simulink model "TemperatureConverter"  (R2024a)
settings: Solver=VariableStepAuto  StartTime=0.0  StopTime=10.0  RelTol=1e-3
values from neighbouring files (symbols this model uses):
  C = input(prompt)    [TemperatureConverter_TrialRun.m]
settings Model: Creator=ammaa  LastModifiedBy=ammaa

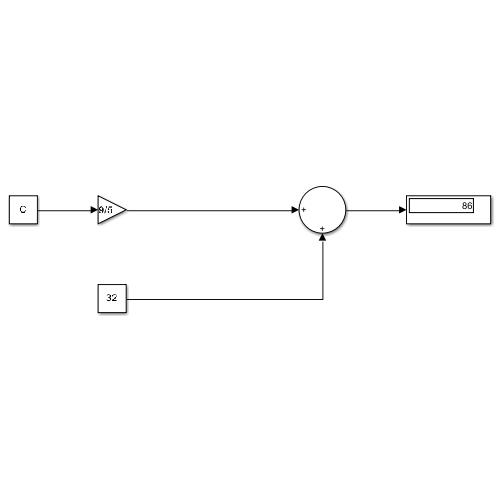
[thumbnail: Simulink's stored preview of the top-level diagram]
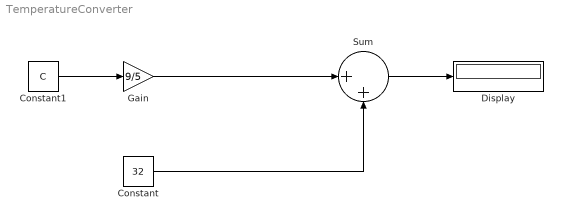
== system TemperatureConverter ==
  Constant : Constant  Value=32
  Constant1 : Constant  Value=C
  Display : Display
  Gain : Gain  Gain=9/5
  Sum : Sum  Inputs=|++
  wires:
  Gain/1 -> Sum/1
  Constant/1 -> Sum/2
  Sum/1 -> Display/1
  Constant1/1 -> Gain/1
